simulink model "par_Filter_OhneC"  (R2019b)
settings: Solver=ode23t  StartTime=0.0  StopTime=1  RelTol=1e-3
model workspace (MAT data in the model file):
  a = 0
libraries: fl_lib x24, nesl_utility x9, ee_lib x6
settings Model: Creator=korschunov  LastModifiedBy=korschunov

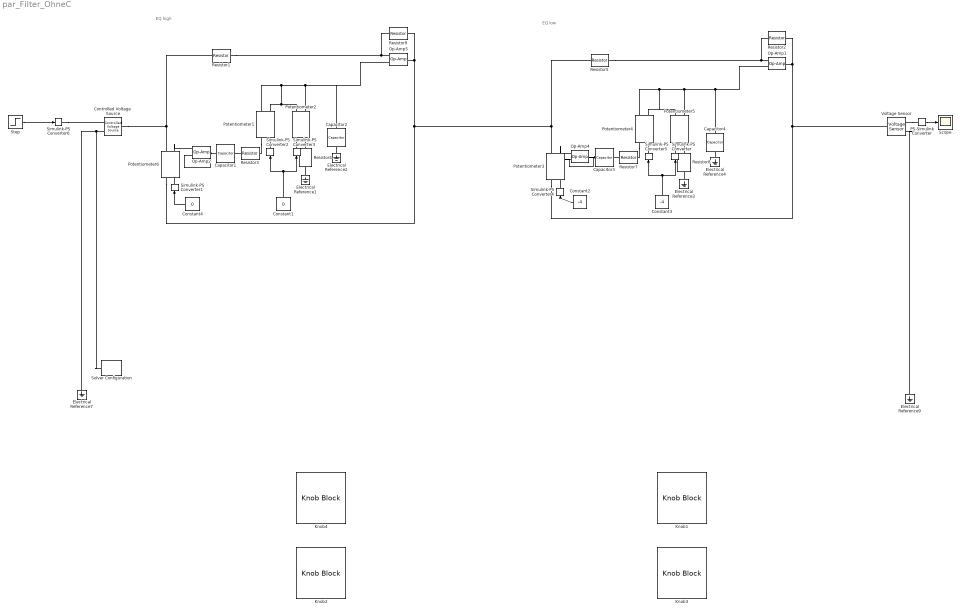
== system par_Filter_OhneC ==
  note: EQ low
  note: EQ high
  Capacitor1 : fl_lib/Electrical/Electrical Elements/Capacitor  c=3.3 nF  r=0 Ohm  g=0 1/Ohm  i_specify=off  i_priority=None  i=0 A  i_nominal_specify=off  i_nominal_unit=A  i_nominal_value=1  v_specify=off  v_priority=None  v=0 V  v_nominal_specify=off  v_nominal_unit=V  v_nominal_value=1  vc_specify=off  vc_priority=High  vc=0 V  vc_nominal_specify=off  vc_nominal_unit=V  vc_nominal_value=1
  Capacitor2 : fl_lib/Electrical/Electrical Elements/Capacitor  c=470 pF  r=0 Ohm  g=0 1/Ohm  i_specify=off  i_priority=None  i=0 A  i_nominal_specify=off  i_nominal_unit=A  i_nominal_value=1  v_specify=off  v_priority=None  v=0 V  v_nominal_specify=off  v_nominal_unit=V  v_nominal_value=1  vc_specify=off  vc_priority=High  vc=0 V  vc_nominal_specify=off  vc_nominal_unit=V  vc_nominal_value=1
  Capacitor3 : fl_lib/Electrical/Electrical Elements/Capacitor  c=100 nF  r=0 Ohm  g=0 1/Ohm  i_specify=off  i_priority=None  i=0 A  i_nominal_specify=off  i_nominal_unit=A  i_nominal_value=1  v_specify=off  v_priority=None  v=0 V  v_nominal_specify=off  v_nominal_unit=V  v_nominal_value=1  vc_specify=off  vc_priority=High  vc=0 V  vc_nominal_specify=off  vc_nominal_unit=V  vc_nominal_value=1
  Capacitor4 : fl_lib/Electrical/Electrical Elements/Capacitor  c=15 nF  r=0 Ohm  g=0 1/Ohm  i_specify=off  i_priority=None  i=0 A  i_nominal_specify=off  i_nominal_unit=A  i_nominal_value=1  v_specify=off  v_priority=None  v=0 V  v_nominal_specify=off  v_nominal_unit=V  v_nominal_value=1  vc_specify=off  vc_priority=High  vc=0 V  vc_nominal_specify=off  vc_nominal_unit=V  vc_nominal_value=1
  Constant1 : Constant  Value=0
  Constant2 : Constant  Value=-4
  Constant3 : Constant  Value=-4
  Constant4 : Constant  Value=0
  Controlled Voltage Source : fl_lib/Electrical/Electrical Sources/Controlled Voltage Source
  Electrical Reference{1..4,7,9} (6 alike) : fl_lib/Electrical/Electrical Elements/Electrical Reference
  Knob{1..4} (4 alike) : KnobBlock  ScaleMin=-4  ScaleMax=+4
  Op-Amp{1..2,4..5} (4 alike) : fl_lib/Electrical/Electrical Elements/Op-Amp  outI_specify=off  outI_priority=None  outI=0 A  outI_nominal_specify=off  outI_nominal_unit=A  outI_nominal_value=1
  PS-Simulink Converter : nesl_utility/PS-Simulink Converter  PhysicalDomain=network_engine_domain  SubClassName=ps_output  LeftPortType=input  RightPortType=output  PseudoPeriodic=off  Frequencies=[]  Unit=inherit  AffineConversion=off
  Potentiometer{1..2,4..5} (4 alike) : ee_lib/Passive/Potentiometer  R0=100 kOhm  Rw=1 Ohm  Rcenter=200 Ohm  xmin=-4  xmax=+4  Taper=1  Gradient=1
      settings: SourceProductName=Simscape Electrical  SourceProductBaseCode=PS  InternalSimscapePortConfiguration="{\"Bottom\":[],\"Left\":[{\"id\":\"pinL\",\"label\":\"L\",\"type\":\"foundation.electrical.electrical\"},{\"id\":\"W\",\"label\":\"W\",\"type\":\"foundation.electrical.electrical\"}],\"Right\":[{\"id\":\"pinR\",\"label\":\"R\",\"type\":\"foundation.electrical.electrical\"},{\"id\":\"x\",\"label\":\"x\",\"type\":\"input\"}],\"Top\":[]}"
  Potentiometer3 : ee_lib/Passive/Potentiometer  R0=47 kOhm  Rw=1 Ohm  Rcenter=200 Ohm  xmin=-4  xmax=+4  Taper=1  Gradient=1
      settings: SourceProductName=Simscape Electrical  SourceProductBaseCode=PS  InternalSimscapePortConfiguration="{\"Bottom\":[],\"Left\":[{\"id\":\"pinL\",\"label\":\"L\",\"type\":\"foundation.electrical.electrical\"},{\"id\":\"W\",\"label\":\"W\",\"type\":\"foundation.electrical.electrical\"}],\"Right\":[{\"id\":\"pinR\",\"label\":\"R\",\"type\":\"foundation.electrical.electrical\"},{\"id\":\"x\",\"label\":\"x\",\"type\":\"input\"}],\"Top\":[]}"
  Potentiometer6 : ee_lib/Passive/Potentiometer  R0=47 kOhm  Rw=1 Ohm  Rcenter=200 Ohm  xmin=-4  xmax=+4  Taper=1  Gradient=1
      settings: SourceProductName=Simscape Electrical  SourceProductBaseCode=PS  InternalSimscapePortConfiguration="{\"Bottom\":[],\"Left\":[{\"id\":\"pinL\",\"label\":\"L\",\"type\":\"foundation.electrical.electrical\"},{\"id\":\"W\",\"label\":\"W\",\"type\":\"foundation.electrical.electrical\"}],\"Right\":[{\"id\":\"pinR\",\"label\":\"R\",\"type\":\"foundation.electrical.electrical\"},{\"id\":\"x\",\"label\":\"x\",\"type\":\"input\"}],\"Top\":[]}"
  Resistor{1..2,5,9} (4 alike) : fl_lib/Electrical/Electrical Elements/Resistor  R=22 kOhm  i_specify=off  i_priority=None  i=0 A  i_nominal_specify=off  i_nominal_unit=A  i_nominal_value=1  v_specify=off  v_priority=None  v=0 V  v_nominal_specify=off  v_nominal_unit=V  v_nominal_value=1
  Resistor{3..4,7..8} (4 alike) : fl_lib/Electrical/Electrical Elements/Resistor  R=6.8 kOhm  i_specify=off  i_priority=None  i=0 A  i_nominal_specify=off  i_nominal_unit=A  i_nominal_value=1  v_specify=off  v_priority=None  v=0 V  v_nominal_specify=off  v_nominal_unit=V  v_nominal_value=1
  Scope : Scope
  Simulink-PS Converter{,1..4,6} (6 alike) : nesl_utility/Simulink-PS Converter  PhysicalDomain=network_engine_domain  SubClassName=ps_input  LeftPortType=input  RightPortType=output  PseudoPeriodic=off  Frequencies=[]  NoiseDistribution=none  NoiseParameters=[]  Unit=1  AffineConversion=off  FilteringAndDerivatives=provide  SimscapeFilterOrder=1  InputFilterTimeConstant=0.001  UdotUserProvided=0
  Simulink-PS Converter5 : nesl_utility/Simulink-PS Converter  PhysicalDomain=network_engine_domain  SubClassName=ps_input  LeftPortType=input  RightPortType=output  PseudoPeriodic=off  Frequencies=[]  NoiseDistribution=none  NoiseParameters=[]  Unit=1  AffineConversion=on  FilteringAndDerivatives=provide  SimscapeFilterOrder=1  InputFilterTimeConstant=0.001  UdotUserProvided=0
  Solver Configuration : nesl_utility/Solver Configuration  PhysicalDomain=network_engine_domain  SubClassName=solver  LeftPortType=input  RightPortType=generic  Tones=[]  Harmonics=[]  SimulateNoise=off  Profile=off  UseLocalSampling=off  EnableSwitchedLinearOptims=on  FrequencyDomain=off  UseCCode=off  RelTol=0.001  AbsTol=1e-06  MinStep=1e-09  ToWorkspace=off  RevertToSquareIcSolve=off  NumHomotopyIterations=100  PhasorMode=off  PhasorModeNumHarmonics=1  DoDC=off  ResidualTolerance=1e-09  UseLocalSolver=off  LocalSolverChoice=NE_BACKWARD_EULER_ADVANCER  LocalSolverSampleTime=0.001  DoFixedCost=off  MaxNonlinIter=3  MaxModeIter=2  LinearAlgebra=auto  EquationFormulation=NE_TIME_EF  DelaysMemoryBudget=1024  AutomaticFiltering=on  FilteringTimeConstant=0.001  PartitionStorageMethod=AS_NEEDED  PartitionMemoryBudget=1024  PartitionMethod=ROBUST
  Step : Step  SampleTime=0
  Voltage Sensor : fl_lib/Electrical/Electrical Sensors/Voltage Sensor
  wires:
  Step/1 -> Simulink-PS Converter6/1
  PS-Simulink Converter/1 -> Scope/1
  Constant4/1 -> Simulink-PS Converter1/1
  Constant1/1 -> Simulink-PS Converter3/1, Simulink-PS Converter2/1
  Constant2/1 -> Simulink-PS Converter4/1
  Constant3/1 -> Simulink-PS Converter/1, Simulink-PS Converter5/1
  connections:
  Simulink-PS Converter6/RConn1 -- Controlled Voltage Source/RConn1
  Electrical Reference7/LConn1 -- Controlled Voltage Source/RConn2 -- Solver Configuration/RConn1
  Voltage Sensor/RConn2 -- Electrical Reference9/LConn1
  Voltage Sensor/RConn1 -- PS-Simulink Converter/LConn1
  Resistor1/RConn1 -- Resistor9/RConn1 -- Op-Amp5/LConn2
  Simulink-PS Converter1/RConn1 -- Potentiometer6/RConn2
  Potentiometer6/LConn2 -- Op-Amp2/LConn1
  Resistor3/LConn1 -- Capacitor1/RConn1
  Potentiometer2/RConn2 -- Simulink-PS Converter3/RConn1
  Potentiometer1/RConn1 -- Resistor3/RConn1
  Potentiometer2/RConn1 -- Resistor4/LConn1
  Potentiometer1/LConn2 -- Potentiometer2/LConn2 -- Potentiometer1/LConn1 -- Potentiometer2/LConn1 -- Op-Amp5/LConn1 -- Capacitor2/LConn1
  Electrical Reference2/LConn1 -- Capacitor2/RConn1
  Simulink-PS Converter2/RConn1 -- Potentiometer1/RConn2
  Electrical Reference1/LConn1 -- Resistor4/RConn1
  Op-Amp2/LConn2 -- Op-Amp2/RConn1 -- Capacitor1/LConn1
  Potentiometer6/LConn1 -- Resistor1/LConn1 -- Controlled Voltage Source/LConn1
  Potentiometer3/LConn2 -- Op-Amp4/LConn1
  Simulink-PS Converter4/RConn1 -- Potentiometer3/RConn2
  Electrical Reference4/LConn1 -- Capacitor4/RConn1
  Resistor7/LConn1 -- Capacitor3/RConn1
  Simulink-PS Converter5/RConn1 -- Potentiometer4/RConn2
  Potentiometer6/RConn1 -- Resistor5/LConn1 -- Potentiometer3/LConn1 -- Resistor9/LConn1 -- Op-Amp5/RConn1
  Capacitor4/LConn1 -- Op-Amp1/LConn1 -- Potentiometer5/LConn1 -- Potentiometer4/LConn1 -- Potentiometer4/LConn2 -- Potentiometer5/LConn2
  Op-Amp4/RConn1 -- Op-Amp4/LConn2 -- Capacitor3/LConn1
  Resistor5/RConn1 -- Resistor2/RConn1 -- Op-Amp1/LConn2
  Electrical Reference3/LConn1 -- Resistor8/RConn1
  Potentiometer5/RConn1 -- Resistor8/LConn1
  Simulink-PS Converter/RConn1 -- Potentiometer5/RConn2
  Potentiometer3/RConn1 -- Resistor2/LConn1 -- Op-Amp1/RConn1 -- Voltage Sensor/LConn1
  Potentiometer4/RConn1 -- Resistor7/RConn1
